simulink model "Zustandsregelung_mit_I_Regelung_linear"  (R2021b)
settings: Solver=FixedStepAuto  StartTime=0.0  StopTime=10  FixedStep=1/1e4  RelTol=1e-3
undefined symbols (not defined in the file): A, B, C, d, delta_y_ref_I_Reg, x_Ruhe
settings Model: Creator=basti  LastModifiedBy=basti

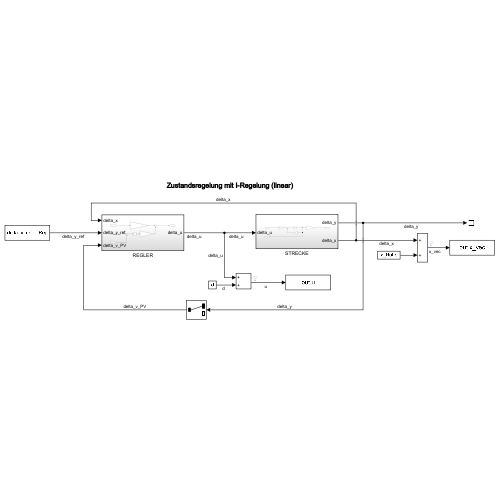
[thumbnail: Simulink's stored preview of the top-level diagram]
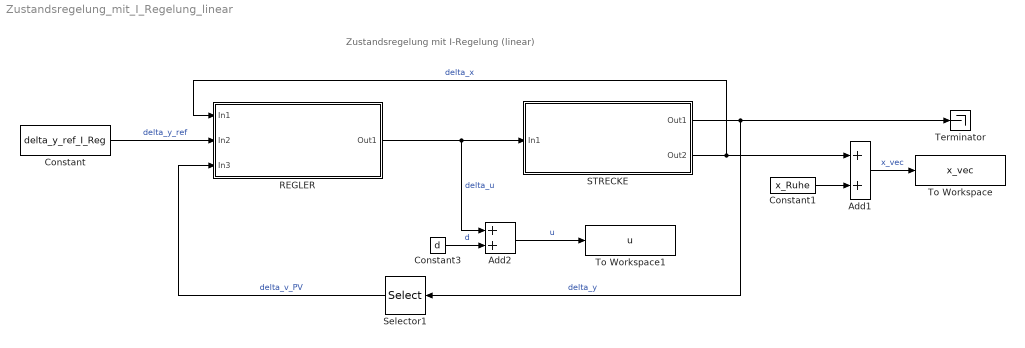
== system Zustandsregelung_mit_I_Regelung_linear ==
  note: Zustandsregelung mit I-Regelung (linear)
  Add1 : Sum
  Add2 : Sum
  Constant : Constant  Value=delta_y_ref_I_Reg
  Constant1 : Constant  Value=x_Ruhe
  Constant3 : Constant  Value=d
  REGLER : Subsystem
  STRECKE : Subsystem
  Selector1 : Selector  InputPortWidth=2  IndexOptions=Index vector (dialog)  Indices=1  OutputSizes=1
  Terminator : Terminator
  To Workspace : ToWorkspace  VariableName=x_vec  SaveFormat=Timeseries  SampleTime=-1
  To Workspace1 : ToWorkspace  VariableName=u  SaveFormat=Timeseries  SampleTime=-1
  wires:
  STRECKE/1(Out1) -> Selector1/1, Terminator/1  "delta_y"
  Constant/1 -> REGLER/2(In2)  "delta_y_ref"
  Selector1/1 -> REGLER/3(In3)  "delta_v_PV"
  Constant1/1 -> Add1/2
  Add1/1 -> To Workspace/1  "x_vec"
  STRECKE/2(Out2) -> Add1/1, REGLER/1(In1)  "delta_x"
  Constant3/1 -> Add2/2  "d"
  REGLER/1(Out1) -> Add2/1, STRECKE/1(In1)  "delta_u"
  Add2/1 -> To Workspace1/1  "u"

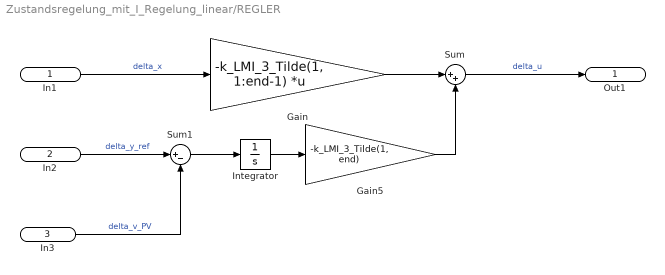
== system Zustandsregelung_mit_I_Regelung_linear/REGLER ==
  In1 : Inport
  In2 : Inport  Port=2
  In3 : Inport  Port=3
  Gain : Gain  Gain=-k_LMI_3_Tilde(1, 1:end-1)  Multiplication=Matrix(K*u) (u vector)
  Gain5 : Gain  Gain=-k_LMI_3_Tilde(1, end)
  Integrator : Integrator
  Sum : Sum  Inputs=|++
  Sum1 : Sum  Inputs=|+-
  Out1 : Outport
  wires:
  Gain/1 -> Sum/1
  In1/1 -> Gain/1  "delta_x"
  Sum/1 -> Out1/1  "delta_u"
  In2/1 -> Sum1/1  "delta_y_ref"
  In3/1 -> Sum1/2  "delta_v_PV"
  Integrator/1 -> Gain5/1
  Sum1/1 -> Integrator/1
  Gain5/1 -> Sum/2

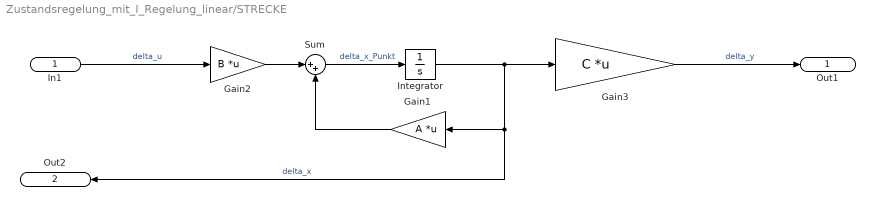
== system Zustandsregelung_mit_I_Regelung_linear/STRECKE ==
  In1 : Inport
  Gain1 : Gain  Gain=A  Multiplication=Matrix(K*u) (u vector)
  Gain2 : Gain  Gain=B  Multiplication=Matrix(K*u) (u vector)
  Gain3 : Gain  Gain=C  Multiplication=Matrix(K*u) (u vector)
  Integrator : Integrator
  Sum : Sum  Inputs=|++
  Out1 : Outport
  Out2 : Outport  Port=2
  wires:
  Gain1/1 -> Sum/2
  Gain3/1 -> Out1/1  "delta_y"
  Sum/1 -> Integrator/1  "delta_x_Punkt"
  Integrator/1 -> Out2/1, Gain1/1, Gain3/1  "delta_x"
  Gain2/1 -> Sum/1
  In1/1 -> Gain2/1  "delta_u"
